simulink model "Model1_Clarke_Park"  (R2021b)
settings: Solver=ode45  StartTime=0.0  StopTime=100  MaxStep=1e-4  RelTol=1e-4  EnableMultiTasking=on
libraries: spspowerguiLib x1
settings Model: Creator=edu  LastModifiedBy=eprieto
settings SolverCC: AlgebraicLoopSolver=TrustRegion
settings DataIOCC: LimitDataPoints=on  SaveFormat=Array  SignalLoggingSaveFormat=ModelDataLogs  ReturnWorkspaceOutputs=off
settings OptimizationCC: ExpressionDepthLimit=2147483647  LifeSpan=inf
settings DebuggingCC: UnderspecifiedInitializationDetection=Classic  MergeDetectMultiDrivingBlocksExec=none  SolverPrmCheckMsg=warning  MultiTaskDSMMsg=warning  MultiTaskCondExecSysMsg=none  FcnCallInpInsideContextMsg=warning  StateNameClashWarn=warning  SFUnexpectedBacktrackingDiag=warning  SFNoUnconditionalDefaultTransitionDiag=warning  SFExecutionAtInitializationDiag=none  SFMachineParentedDataDiag=warning  ArithmeticOperatorsInVariantConditions=warning
settings HardwareCC: ProdBitPerPointer=32  ProdBitPerSizeT=32  ProdBitPerPtrDiffT=32  ProdLargestAtomicFloat=None  ProdIntDivRoundTo=Undefined  ProdEndianess=Unspecified  ProdWordSize=32  ProdHWDeviceType=32-bit Generic
settings ModelReferenceCC: PropagateSignalLabelsOutOfModel=off
settings SFSimCC: SimUseLocalCustomCode=off  CustomCodeUndefinedFunction=UseInterfaceOnly
settings RTWCC: RTWUseLocalCustomCode=off
settings CodeAppCC: StateflowObjectComments=on
settings GRTTargetCC: TargetLangStandard=C89/C90 (ANSI)  CombineOutputUpdateFcns=off  GRTInterface=on
settings ConfigComp: CovMetricSettings=dw  CovSaveCumulativeToWorkspaceVar=on  CovSaveSingleToWorkspaceVar=on  CovExternalEMLEnable=off
settings SimscapeCC: SimscapeNormalizeSystem=off
settings ConfigurationSet: Description=SimMechanics 2G

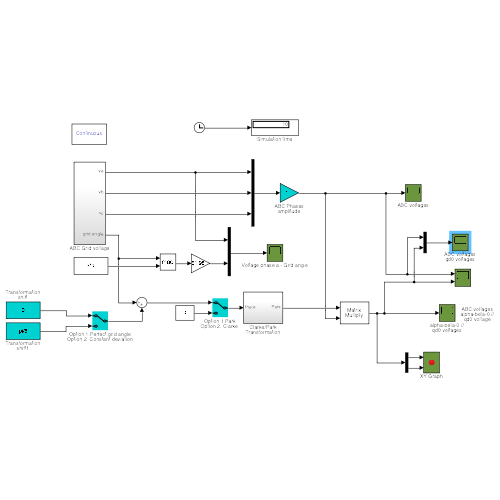
[thumbnail: Simulink's stored preview of the top-level diagram]
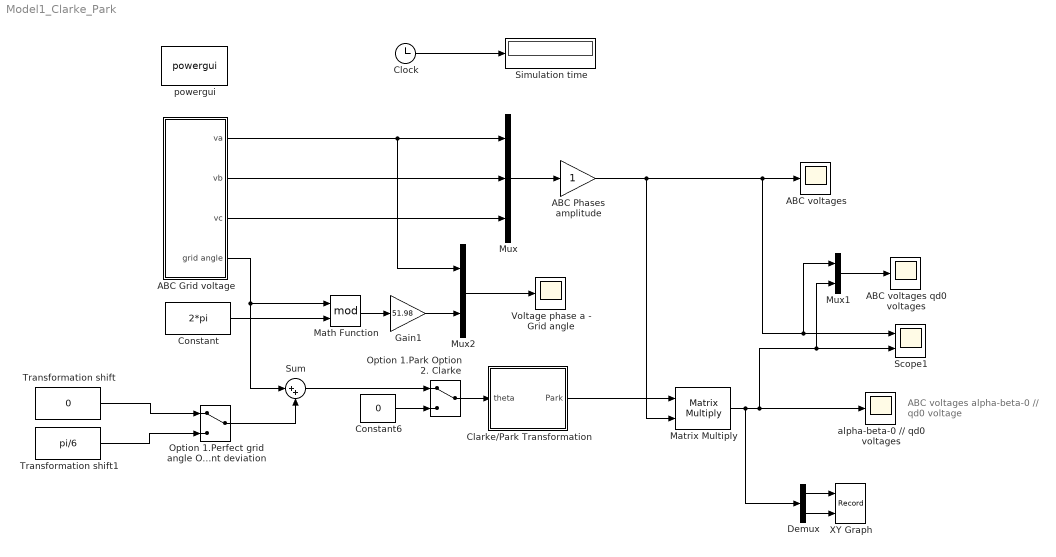
== system Model1_Clarke_Park ==
  note: ABC voltages
      | alpha-beta-0 //
      | qd0 voltage
  "ABC Grid voltage " : Subsystem
  ABC Phases amplitude : Gain
  ABC voltages : Scope
  ABC voltages qd0 voltages : Scope
  Clarke/Park Transformation : Subsystem
  Clock : Clock
  Constant : Constant  Value=2*pi
  Constant6 : Constant  Value=0
  Demux : Demux  Outputs=2
  Gain1 : Gain  Gain=51.98
  Math Function : Math  Operator=mod  SignedPower=on  SaturateOnIntegerOverflow=on
  Matrix Multiply : Product  Multiplication=Matrix(*)
  Mux : Mux  Inputs=3
  Mux1 : Mux  Inputs=2
  Mux2 : Mux  Inputs=2
  "Option 1.Park Option 2. Clarke " : ManualSwitch
  Option 1.Perfect grid angle Option 2. Constant deviation : ManualSwitch
  Scope1 : Scope  NumInputPorts=2
  Simulation time : Display
  Sum : Sum  Inputs=|++
  Transformation shift : Constant  Value=0
  Transformation shift1 : Constant  Value=pi/6
  Voltage phase a - Grid angle : Scope
  XY Graph : Record  FileSettingsInternal="{\"entries\":[{\"content\":{\"excelSettings\":{\"content\":{},\"type\":\"Streamout.ExcelSettings\"}},\"type\":\"Streamout.FileSettingStorage\",\"uuid\":\"46808af6-af5b-4f47-8ec5-4aefbb458854\"}],\"packageUris\":[\"http://schema.mathworks.com/mf0/streamout_blocks/R2020a\"],\"version\":\"1.0\"}"  Layout=[1 1]  SignalsInternal="{\"entries\":[{\"content\":{\"signals\":[{\"content\":{\"blockPath\":[\"Model1_Clarke_Park_12/XY Graph\"],\"channel\":[],\"dimensions\":[1],\"domain\":\"Model1_Clarke_Park_12/XY Graph\",\"lineColor\":\"#a2142f\",\"plots\":[1],\"port\":1,\"sid\":[\"\"],\"signalID\":28,\"signalName\":\"Demux:1\"},\"type\":\"RecordBlkView.Signal\",\"uuid\":\"8c3e991a-e888-4b3b-9b8b-4e4bda5e29b2\"},{\"content\":{\"blockPath\":[\"Model1_Clarke_Park_12/XY Graph\"],\"channel\":[],\"dimensions\":[1],\"domain\":\"Model1_Clarke_Park_12/XY Graph\",\"lineColor\":\"#139fff\",\"plots\":[1],\"port\":2,\"sid\":[\"\"],\"signalID\":32,\"signalName\":\"Demux:2\"},\"type\":\"RecordBlkView.Signal\",\"uuid\":\"df96f0c8-2096-4bfd-a5c5-dfbd894b470f\"}]},\"type\":\"RecordBlkView.InputSignals\",\"uuid\":\"14d7049d-80ef-48d4-ab71-f65b6a0dab3c\"}],\"packageUris\":[\"http://schema.mathworks.com/mf0/streamout_blocks/R2020a\"],\"version\":\"1.0\"}"  VisualizationBindings="{\"xyplotplugin\":{\"info\":[{\"series\":[{\"bindingParametersList\":[{\"parameter\":\"X-Axis\",\"signalID\":28,\"signalName\":\"Demux:1\"},{\"parameter\":\"Y-Axis\",\"signalID\":32,\"signalName\":\"Demux:2\"}],\"seriesID\":48390}],\"subplotID\":1}]}}"  CompatibilityTag=XY  st=-1
  alpha-beta-0 // qd0 voltages : Scope
  powergui : spspowerguiLib/powergui  Priority=1  SimulationMode=Continuous  SampleTime=50e-6  frequency=60  Iterations=50  frequencyindice=0  Pbase=100e6  ErrMax=1e-4  UnitsV=kV  UnitsW=MW  buscounter=0  FunctionMessages=off  echomessages=off  EnableUseOfTLC=off  CurrentSourceSwitches=off  DisableSnubberDevices=off  DisableRonSwitches=off  DisableVfSwitches=off  DisplayEquations=off  AutomaticDiscreteSolvers=off  SolverType=Tustin  Interpol=off  ExternalGateDelay=off  methode=off  Ts=0  x0status=blocks  SPID=off  SwTol=0  HookPort=off  NonlinearTolerance=1e-4  nMaxIteration=100  ContinueOnMaxIteration=off  RestoreLinks=warning  ResistiveCurrentMeasurement=off  Frange=[0:2:500]  Ylog=off  Xlog=on  ShowGrid=off  save=off  variable=ZData  structure=0  ZoomFFT=off  StartTime=0.0  cycles=1  DisplayStyle=1  fundamental=60  FreqAxis=off  MaxFrequency=1000  frequencyindicesteady=1  RmsSteady=1  display=off
  wires:
  Mux/1 -> ABC Phases amplitude/1
  Clock/1 -> Simulation time/1
  Clarke/Park Transformation/1(Park) -> Matrix Multiply/1
  Matrix Multiply/1 -> Demux/1, alpha-beta-0 // qd0 voltages/1, Mux1/2, Scope1/2
  Mux1/1 -> ABC voltages qd0 voltages/1
  "ABC Grid voltage "/1(va) -> Mux2/1, Mux/1
  "ABC Grid voltage "/2(vb) -> Mux/2
  "ABC Grid voltage "/3(vc) -> Mux/3
  Mux2/1 -> Voltage phase a - Grid angle/1
  Math Function/1 -> Gain1/1
  Constant/1 -> Math Function/2
  Gain1/1 -> Mux2/2
  "ABC Grid voltage "/4(grid angle) -> Sum/1, Math Function/1
  "Option 1.Park Option 2. Clarke "/1 -> Clarke/Park Transformation/1(theta)
  Constant6/1 -> "Option 1.Park Option 2. Clarke "/2
  Sum/1 -> "Option 1.Park Option 2. Clarke "/1
  Option 1.Perfect grid angle Option 2. Constant deviation/1 -> Sum/2
  Demux/1 -> XY Graph/1
  Demux/2 -> XY Graph/2
  ABC Phases amplitude/1 -> ABC voltages/1, Mux1/1, Scope1/1, Matrix Multiply/2
  Transformation shift/1 -> Option 1.Perfect grid angle Option 2. Constant deviation/1
  Transformation shift1/1 -> Option 1.Perfect grid angle Option 2. Constant deviation/2

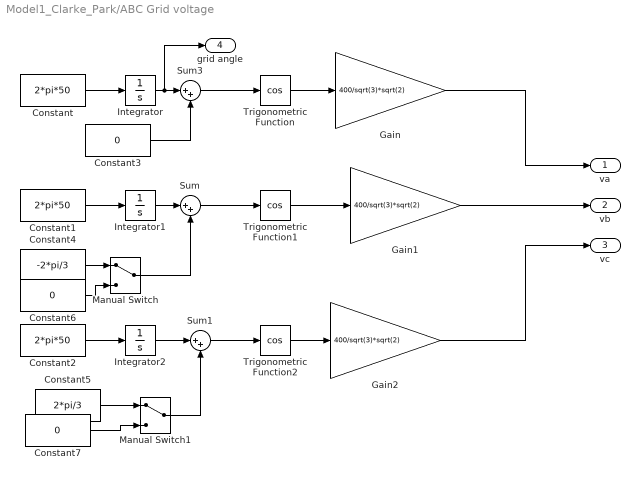
== system Model1_Clarke_Park/ABC Grid voltage  ==
  Constant : Constant  Value=2*pi*50
  Constant1 : Constant  Value=2*pi*50
  Constant2 : Constant  Value=2*pi*50
  Constant3 : Constant  Value=0
  Constant4 : Constant  Value=-2*pi/3
  Constant5 : Constant  Value=2*pi/3
  Constant6 : Constant  Value=0
  Constant7 : Constant  Value=0
  Gain : Gain  Gain=400/sqrt(3)*sqrt(2)
  Gain1 : Gain  Gain=400/sqrt(3)*sqrt(2)
  Gain2 : Gain  Gain=400/sqrt(3)*sqrt(2)
  Integrator : Integrator
  Integrator1 : Integrator
  Integrator2 : Integrator
  Manual Switch : ManualSwitch
  Manual Switch1 : ManualSwitch
  Sum : Sum  Inputs=|++
  Sum1 : Sum  Inputs=|++
  Sum3 : Sum  Inputs=|++
  Trigonometric Function : Trigonometry  Operator=cos
  Trigonometric Function1 : Trigonometry  Operator=cos
  Trigonometric Function2 : Trigonometry  Operator=cos
  va : Outport
  vb : Outport  Port=2
  vc : Outport  Port=3
  grid angle : Outport  Port=4
  wires:
  Constant2/1 -> Integrator2/1
  Integrator2/1 -> Sum1/1
  Gain2/1 -> vc/1
  Sum1/1 -> Trigonometric Function2/1
  Sum3/1 -> Trigonometric Function/1
  Integrator/1 -> grid angle/1, Sum3/1
  Manual Switch1/1 -> Sum1/2
  Manual Switch/1 -> Sum/2
  Integrator1/1 -> Sum/1
  Trigonometric Function/1 -> Gain/1
  Gain/1 -> va/1
  Constant1/1 -> Integrator1/1
  Trigonometric Function2/1 -> Gain2/1
  Constant/1 -> Integrator/1
  Constant3/1 -> Sum3/2
  Trigonometric Function1/1 -> Gain1/1
  Gain1/1 -> vb/1
  Sum/1 -> Trigonometric Function1/1
  Constant4/1 -> Manual Switch/1
  Constant6/1 -> Manual Switch/2
  Constant5/1 -> Manual Switch1/1
  Constant7/1 -> Manual Switch1/2

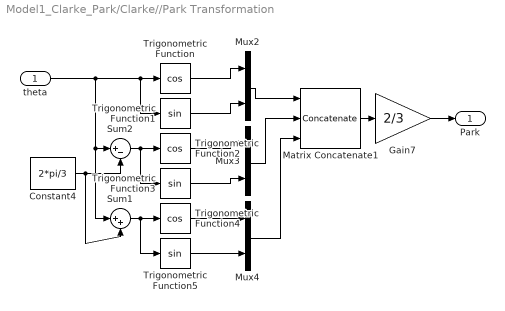
== system Model1_Clarke_Park/Clarke//Park Transformation ==
  theta : Inport  PortDimensions=1
  Constant4 : Constant  Value=2*pi/3  SampleTime=-1
  Gain7 : Gain  Gain=2/3
  Matrix Concatenate1 : Concatenate  NumInputs=3  Mode=Multidimensional array  ConcatenateDimension=2
  Mux2 : Mux  Inputs=2
  Mux3 : Mux  Inputs=2
  Mux4 : Mux  Inputs=2
  Sum1 : Sum  Inputs=|++
  Sum2 : Sum  Inputs=|+-
  Trigonometric Function : Trigonometry  Operator=cos
  Trigonometric Function1 : Trigonometry
  Trigonometric Function2 : Trigonometry  Operator=cos
  Trigonometric Function3 : Trigonometry
  Trigonometric Function4 : Trigonometry  Operator=cos
  Trigonometric Function5 : Trigonometry
  Park : Outport
  wires:
  theta/1 -> Sum1/1, Sum2/1, Trigonometric Function/1, Trigonometric Function1/1
  Sum2/1 -> Trigonometric Function2/1, Trigonometric Function3/1
  Sum1/1 -> Trigonometric Function4/1, Trigonometric Function5/1
  Constant4/1 -> Sum2/2, Sum1/2
  Trigonometric Function/1 -> Mux2/1
  Trigonometric Function1/1 -> Mux2/2
  Trigonometric Function2/1 -> Mux3/1
  Trigonometric Function3/1 -> Mux3/2
  Trigonometric Function4/1 -> Mux4/1
  Trigonometric Function5/1 -> Mux4/2
  Mux2/1 -> Matrix Concatenate1/1
  Mux3/1 -> Matrix Concatenate1/2
  Mux4/1 -> Matrix Concatenate1/3
  Matrix Concatenate1/1 -> Gain7/1
  Gain7/1 -> Park/1
